simulink model "Final10"  (R2020a)
settings: Solver=VariableStepAuto  StartTime=0.0  StopTime=2  RelTol=1e-3
libraries: commanapbnd3 x6, dsparch4 x3, dspsrcs4 x3, commchan3 x1
settings Model: Creator=Egor  LastModifiedBy=Egor

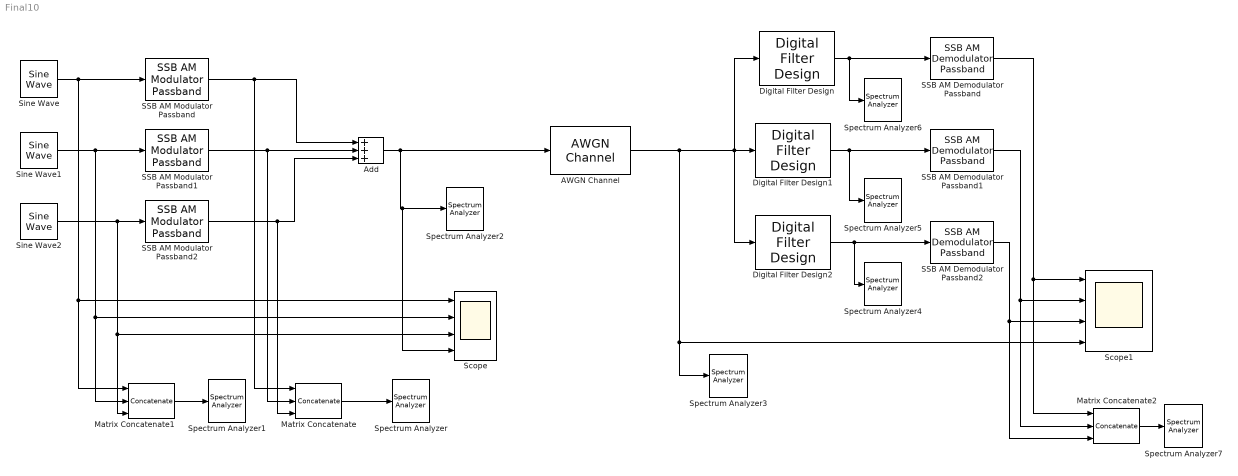
== system Final10 ==
  AWGN Channel : commchan3/AWGN Channel  InputProcessing=Columns as channels (frame based)  seed=67  noiseMode="Signal to noise ratio  (Eb/No)"  EbNodB=10  EsNodB=10  SNRdB=10  bitsPerSym=1  Ps=1  Tsym=1  variance=1
  Add : Sum  Inputs=+++
  Digital Filter Design : dsparch4/Digital Filter Design  mwdsp_browser_bugfix_var=off
  Digital Filter Design1 : dsparch4/Digital Filter Design  mwdsp_browser_bugfix_var=off
  Digital Filter Design2 : dsparch4/Digital Filter Design  mwdsp_browser_bugfix_var=off
  Matrix Concatenate : Concatenate  NumInputs=3  ConcatenateDimension=2
  Matrix Concatenate1 : Concatenate  NumInputs=3  ConcatenateDimension=2
  Matrix Concatenate2 : Concatenate  NumInputs=3  ConcatenateDimension=2
  SSB AM Demodulator Passband : commanapbnd3/SSB AM Demodulator Passband  Fc=120  Ph=0  method=Butterworth  n=4  cf=100  Rp=0.1  Rs=50
      settings: SourceProductBaseCode=CM
  SSB AM Demodulator Passband1 : commanapbnd3/SSB AM Demodulator Passband  Fc=180  Ph=0  method=Butterworth  n=4  cf=100  Rp=0.1  Rs=50
      settings: SourceProductBaseCode=CM
  SSB AM Demodulator Passband2 : commanapbnd3/SSB AM Demodulator Passband  Fc=240  Ph=0  method=Butterworth  n=4  cf=100  Rp=0.1  Rs=50
      settings: SourceProductBaseCode=CM
  SSB AM Modulator Passband : commanapbnd3/SSB AM Modulator Passband  Fc=120  Ph=0  Sd=Lower  Ho=100
      settings: SourceProductBaseCode=CM
  SSB AM Modulator Passband1 : commanapbnd3/SSB AM Modulator Passband  Fc=180  Ph=0  Sd=Lower  Ho=100
      settings: SourceProductBaseCode=CM
  SSB AM Modulator Passband2 : commanapbnd3/SSB AM Modulator Passband  Fc=240  Ph=0  Sd=Lower  Ho=100
      settings: SourceProductBaseCode=CM
  Scope : Scope  NumInputPorts=4
  Scope1 : Scope  NumInputPorts=4
  Sine Wave : dspsrcs4/Sine Wave  Amplitude=2  Frequency=22  Phase=0  SampleMode=Discrete  OutComplex=Real  CompMethod=Trigonometric fcn  TableSize=Speed  SampleTime=1/1000  SamplesPerFrame=1  ResetState=Restart at time zero  OutputFrames=off  dataType=double  wordLen=16  udDataType=sfix(16)  fracBitsMode=Best precision  numFracBits=15  OutDataTypeStr=double  LastOutDataTypeStr=double
  Sine Wave1 : dspsrcs4/Sine Wave  Amplitude=3  Frequency=44  Phase=0  SampleMode=Discrete  OutComplex=Real  CompMethod=Trigonometric fcn  TableSize=Speed  SampleTime=1/1000  SamplesPerFrame=1  ResetState=Restart at time zero  OutputFrames=off  dataType=double  wordLen=16  udDataType=sfix(16)  fracBitsMode=Best precision  numFracBits=15  OutDataTypeStr=double  LastOutDataTypeStr=double
  Sine Wave2 : dspsrcs4/Sine Wave  Amplitude=5  Frequency=66  Phase=0  SampleMode=Discrete  OutComplex=Real  CompMethod=Trigonometric fcn  TableSize=Speed  SampleTime=1/1000  SamplesPerFrame=1  ResetState=Restart at time zero  OutputFrames=off  dataType=double  wordLen=16  udDataType=sfix(16)  fracBitsMode=Best precision  numFracBits=15  OutDataTypeStr=double  LastOutDataTypeStr=double
  Spectrum Analyzer{,1..7} (8 alike) : SpectrumAnalyzer
  wires:
  SSB AM Modulator Passband1/1 -> Matrix Concatenate/2, Add/2
  Add/1 -> AWGN Channel/1, Scope/4, Spectrum Analyzer2/1
  Sine Wave/1 -> Matrix Concatenate1/1, Scope/1, SSB AM Modulator Passband/1
  Sine Wave1/1 -> Matrix Concatenate1/2, Scope/2, SSB AM Modulator Passband1/1
  Sine Wave2/1 -> Matrix Concatenate1/3, Scope/3, SSB AM Modulator Passband2/1
  SSB AM Modulator Passband2/1 -> Matrix Concatenate/3, Add/3
  SSB AM Modulator Passband/1 -> Matrix Concatenate/1, Add/1
  Matrix Concatenate1/1 -> Spectrum Analyzer1/1
  Matrix Concatenate/1 -> Spectrum Analyzer/1
  Digital Filter Design/1 -> Spectrum Analyzer6/1, SSB AM Demodulator Passband/1
  Digital Filter Design1/1 -> Spectrum Analyzer5/1, SSB AM Demodulator Passband1/1
  Digital Filter Design2/1 -> Spectrum Analyzer4/1, SSB AM Demodulator Passband2/1
  AWGN Channel/1 -> Scope1/4, Spectrum Analyzer3/1, Digital Filter Design2/1, Digital Filter Design/1, Digital Filter Design1/1
  SSB AM Demodulator Passband/1 -> Scope1/1, Matrix Concatenate2/1
  SSB AM Demodulator Passband1/1 -> Scope1/2, Matrix Concatenate2/2
  SSB AM Demodulator Passband2/1 -> Scope1/3, Matrix Concatenate2/3
  Matrix Concatenate2/1 -> Spectrum Analyzer7/1
